simulink model "xz_coordinate_stab_control"  (R2020a)
settings: Solver=VariableStepAuto  StartTime=0.0  StopTime=10.0  RelTol=1e-3
settings Model: Creator=Tamer  LastModifiedBy=Tamer

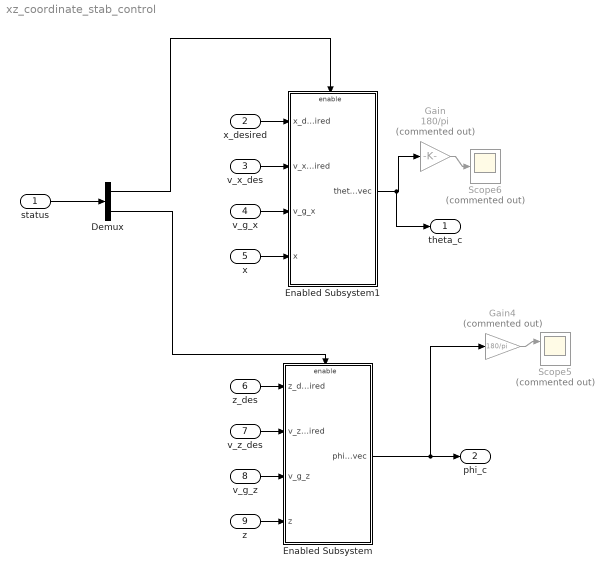
== system xz_coordinate_stab_control ==
  status : Inport
  x_desired : Inport  Port=2
  v_x_des : Inport  Port=3
  v_g_x : Inport  Port=4
  x : Inport  Port=5
  z_des : Inport  Port=6
  v_z_des : Inport  Port=7
  v_g_z : Inport  Port=8
  z : Inport  Port=9
  Demux : Demux  Outputs=2
  Enabled Subsystem : Subsystem  TreatAsAtomicUnit=on
  Enabled Subsystem1 : Subsystem  TreatAsAtomicUnit=on
  Gain : Gain  Commented=on  Gain=180/pi
  Gain4 : Gain  Commented=on  Gain=180/pi
  Scope5 : Scope  Commented=on  NumInputPorts=2
  Scope6 : Scope  Commented=on
  theta_c : Outport
  phi_c : Outport  Port=2
  wires:
  Gain4/1 -> Scope5/1
  Enabled Subsystem/1(phi_c_vec) -> phi_c/1, Gain4/1
  status/1 -> Demux/1
  Demux/1 -> Enabled Subsystem1/Enable
  Demux/2 -> Enabled Subsystem/Enable
  Gain/1 -> Scope6/1
  Enabled Subsystem1/1(theta_c_vec) -> theta_c/1, Gain/1
  x_desired/1 -> Enabled Subsystem1/1(x_desired)
  v_x_des/1 -> Enabled Subsystem1/2(v_x_desired)
  v_g_x/1 -> Enabled Subsystem1/3(v_g_x)
  x/1 -> Enabled Subsystem1/4(x)
  z_des/1 -> Enabled Subsystem/1(z_desired)
  v_z_des/1 -> Enabled Subsystem/2(v_z_desired)
  v_g_z/1 -> Enabled Subsystem/3(v_g_z)
  z/1 -> Enabled Subsystem/4(z)

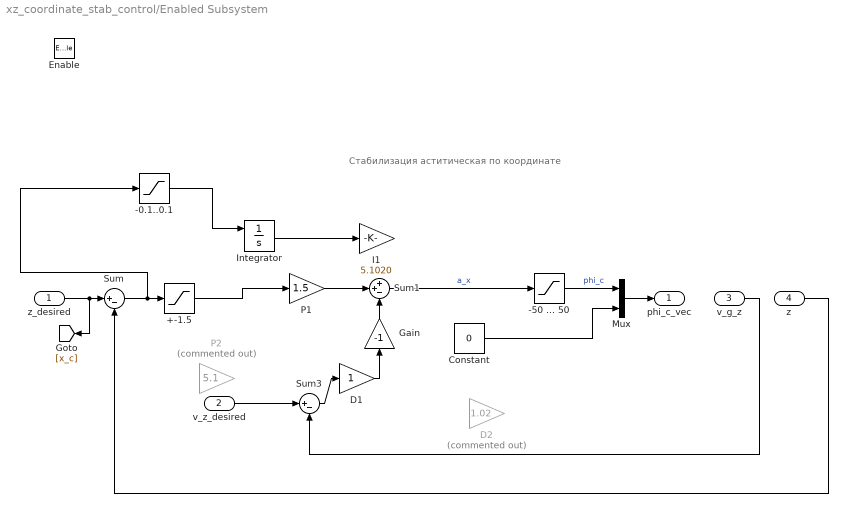
== system xz_coordinate_stab_control/Enabled Subsystem ==
  note: Стабилизация аститическая по координате
  z_desired : Inport
  v_z_desired : Inport  Port=2
  v_g_z : Inport  Port=3
  z : Inport  Port=4
  Enable : EnablePort
  +-1.5 : Saturate  UpperLimit=1.5  LowerLimit=-1.5
  -0.1..0.1 : Saturate  UpperLimit=0.1  LowerLimit=-0.1
  -50 ... 50 : Saturate  UpperLimit=deg2rad(50)  LowerLimit=deg2rad(-50)
  Constant : Constant  Value=0
  D1 : Gain
  D2 : Gain  Commented=on  Gain=1.02
  Gain : Gain  Gain=-1
  I1 : Gain  Gain=5.1020
  Integrator : Integrator  ExternalReset=either
  Mux : Mux  Inputs=2
  P1 : Gain  Gain=1.5
  P2 : Gain  Commented=on  Gain=5.1
  Sum : Sum  Inputs=|+-
  Sum1 : Sum  Inputs=++-
  Sum3 : Sum  Inputs=|+-
  phi_c_vec : Outport
  wires:
  -0.1..0.1/1 -> Integrator/1
  +-1.5/1 -> P1/1
  D1/1 -> Gain/1
  Sum3/1 -> D1/1
  Sum1/1 -> -50 ... 50/1  "a_x"
  Constant/1 -> Mux/2
  Mux/1 -> phi_c_vec/1
  Sum/1 -> -0.1..0.1/1, +-1.5/1
  -50 ... 50/1 -> Mux/1  "phi_c"
  v_g_z/1 -> Sum3/2
  z/1 -> Sum/2
  P1/1 -> Sum1/2
  Gain/1 -> Sum1/3
  z_desired/1 -> [x_c], Sum/1
  v_z_desired/1 -> Sum3/1
  Integrator/1 -> I1/1

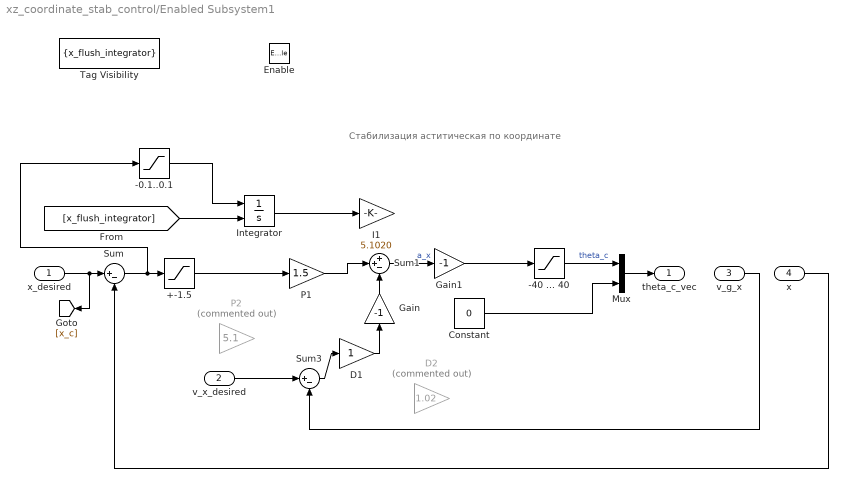
== system xz_coordinate_stab_control/Enabled Subsystem1 ==
  note: Стабилизация аститическая по координате
  x_desired : Inport
  v_x_desired : Inport  Port=2
  v_g_x : Inport  Port=3
  x : Inport  Port=4
  Enable : EnablePort
  +-1.5 : Saturate  UpperLimit=1.5  LowerLimit=-1.5
  -0.1..0.1 : Saturate  UpperLimit=0.1  LowerLimit=-0.1
  -40 ... 40 : Saturate  UpperLimit=deg2rad(50)  LowerLimit=deg2rad(-50)
  Constant : Constant  Value=0
  D1 : Gain
  D2 : Gain  Commented=on  Gain=1.02
  Gain : Gain  Gain=-1
  Gain1 : Gain  Gain=-1
  I1 : Gain  Gain=5.1020
  Integrator : Integrator  ExternalReset=either
  Mux : Mux  Inputs=2
  P1 : Gain  Gain=1.5
  P2 : Gain  Commented=on  Gain=5.1
  Sum : Sum  Inputs=|+-
  Sum1 : Sum  Inputs=++-
  Sum3 : Sum  Inputs=|+-
  Tag Visibility : GotoTagVisibility  GotoTag=x_flush_integrator
  theta_c_vec : Outport
  wires:
  Sum1/1 -> Gain1/1  "a_x"
  Constant/1 -> Mux/2
  Gain1/1 -> -40 ... 40/1
  Integrator/1 -> I1/1
  Mux/1 -> theta_c_vec/1
  +-1.5/1 -> P1/1
  D1/1 -> Gain/1
  x/1 -> Sum/2
  -40 ... 40/1 -> Mux/1  "theta_c"
  x_desired/1 -> [x_c], Sum/1
  [x_flush_integrator] -> Integrator/2
  -0.1..0.1/1 -> Integrator/1
  Gain/1 -> Sum1/3
  Sum/1 -> -0.1..0.1/1, +-1.5/1
  v_g_x/1 -> Sum3/2
  Sum3/1 -> D1/1
  P1/1 -> Sum1/2
  v_x_desired/1 -> Sum3/1
